simulink model "dve_nadrze_rizeni_frekvencni"  (R2016a)
settings: Solver=VariableStepAuto  SolverMode=SingleTasking  StartTime=0.0  StopTime=time  RelTol=1e-3
undefined symbols (not defined in the file): freq
settings Model: Creator=Filip Jašek  LastModifiedBy=Filip Jašek
settings DataIOCC: ReturnWorkspaceOutputs=on
settings DebuggingCC: SFUnexpectedBacktrackingDiag=error  SFNoUnconditionalDefaultTransitionDiag=error
settings SFSimCC: SimUseLocalCustomCode=on
settings RTWCC: RTWUseLocalCustomCode=on
settings GRTTargetCC: TargetLangStandard=C99 (ISO)
settings ConfigComp: CovMetricSettings=dwe  CovHtmlReporting=off  CovSaveCumulativeToWorkspaceVar=off  CovSaveSingleToWorkspaceVar=off  CovExternalEMLEnable=on

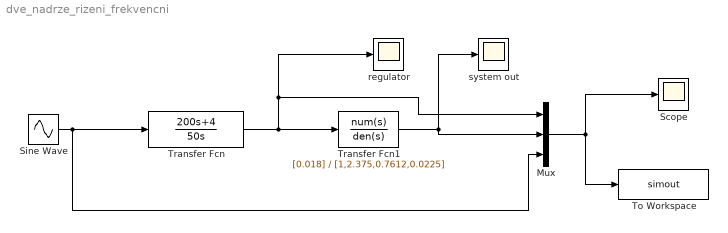
== system dve_nadrze_rizeni_frekvencni ==
  Mux : Mux  Inputs=3
  Scope : Scope
  Sine Wave : Sin  Frequency=freq  SampleTime=0
  To Workspace : ToWorkspace  VariableName=simout  SaveFormat=Timeseries  SampleTime=-1
  Transfer Fcn : TransferFcn  Numerator=[200,4]  Denominator=[50,0]
  Transfer Fcn1 : TransferFcn  Numerator=[0.018]  Denominator=[1,2.375,0.7612,0.0225]
  regulator : Scope
  system out : Scope
  wires:
  Transfer Fcn1/1 -> system out/1, Mux/2
  Sine Wave/1 -> Transfer Fcn/1, Mux/3
  Mux/1 -> To Workspace/1, Scope/1
  Transfer Fcn/1 -> regulator/1, Mux/1, Transfer Fcn1/1
